simulink model "SPGF_FSK_0000_R2020b"  (R2020b)
settings: Solver=ode4  StartTime=0.0  StopTime=1.4  FixedStep=50e-6/50  RelTol=1e-3  EnableMultiTasking=on
undefined symbols (not defined in the file): D11, Delta
libraries: powerlib x2546, powerlib_meascontrol x183, simulink x24
(part 16 of 34)

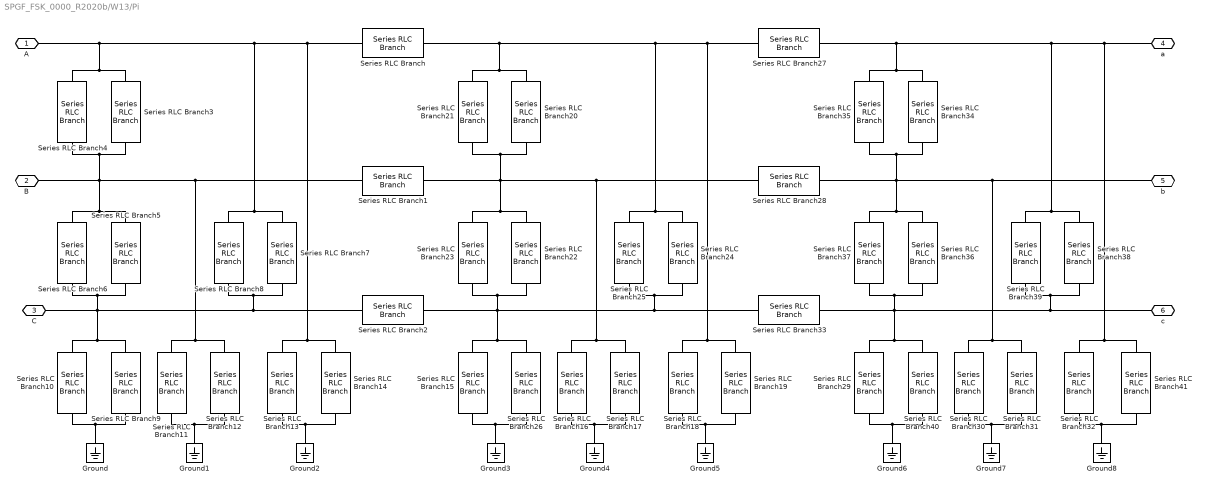
== system SPGF_FSK_0000_R2020b/W13/Pi ==
  Ground{,1..8} (9 alike) : powerlib/Elements/Ground  LConnTagsString=a
  Series RLC Branch{,1..2,27..28,33} (6 alike) : powerlib/Elements/Series RLC Branch  LConnTagsString=__new0  RConnTagsString=__new0  BranchType=RL  Resistance=R/2  Inductance=L/2  SetiL0=off  InitialCurrent=0  Capacitance=1e-6  Setx0=off  InitialVoltage=0  Measurements=None
  Series RLC Branch{10..11,13,29..30,32} (6 alike) : powerlib/Elements/Series RLC Branch  LConnTagsString=__new0  RConnTagsString=__new0  BranchType=R  Resistance=Rfg*4  Inductance=L/2  SetiL0=off  InitialCurrent=0  Capacitance=1e-6  Setx0=off  InitialVoltage=0  Measurements=None
  Series RLC Branch{9,12,14,31,40..41} (6 alike) : powerlib/Elements/Series RLC Branch  LConnTagsString=__new0  RConnTagsString=__new0  BranchType=C  Resistance=R/2  Inductance=L/2  SetiL0=off  InitialCurrent=0  Capacitance=Cfg*0.25  Setx0=off  InitialVoltage=0  Measurements=None
  Series RLC Branch15 : powerlib/Elements/Series RLC Branch  LConnTagsString=__new0  RConnTagsString=__new0  BranchType=R  Resistance=Rfg*2  Inductance=L/2  SetiL0=off  InitialCurrent=0  Capacitance=1e-6  Setx0=off  InitialVoltage=0  Measurements=None
  Series RLC Branch16 : powerlib/Elements/Series RLC Branch  LConnTagsString=__new0  RConnTagsString=__new0  BranchType=R  Resistance=Rfg*2  Inductance=L/2  SetiL0=off  InitialCurrent=0  Capacitance=1e-6  Setx0=off  InitialVoltage=0  Measurements=None
  Series RLC Branch17 : powerlib/Elements/Series RLC Branch  LConnTagsString=__new0  RConnTagsString=__new0  BranchType=C  Resistance=R/2  Inductance=L/2  SetiL0=off  InitialCurrent=0  Capacitance=Cfg*0.5  Setx0=off  InitialVoltage=0  Measurements=None
  Series RLC Branch18 : powerlib/Elements/Series RLC Branch  LConnTagsString=__new0  RConnTagsString=__new0  BranchType=R  Resistance=Rfg*2  Inductance=L/2  SetiL0=off  InitialCurrent=0  Capacitance=1e-6  Setx0=off  InitialVoltage=0  Measurements=None
  Series RLC Branch19 : powerlib/Elements/Series RLC Branch  LConnTagsString=__new0  RConnTagsString=__new0  BranchType=C  Resistance=R/2  Inductance=L/2  SetiL0=off  InitialCurrent=0  Capacitance=Cfg*0.5  Setx0=off  InitialVoltage=0  Measurements=None
  Series RLC Branch20 : powerlib/Elements/Series RLC Branch  LConnTagsString=__new0  RConnTagsString=__new0  BranchType=C  Resistance=R/2  Inductance=L/2  SetiL0=off  InitialCurrent=0  Capacitance=Cmf*0.5  Setx0=off  InitialVoltage=0  Measurements=None
  Series RLC Branch21 : powerlib/Elements/Series RLC Branch  LConnTagsString=__new0  RConnTagsString=__new0  BranchType=R  Resistance=Rmf*2  Inductance=L/2  SetiL0=off  InitialCurrent=0  Capacitance=1e-6  Setx0=off  InitialVoltage=0  Measurements=None
  Series RLC Branch22 : powerlib/Elements/Series RLC Branch  LConnTagsString=__new0  RConnTagsString=__new0  BranchType=C  Resistance=R/2  Inductance=L/2  SetiL0=off  InitialCurrent=0  Capacitance=Cmf*0.5  Setx0=off  InitialVoltage=0  Measurements=None
  Series RLC Branch23 : powerlib/Elements/Series RLC Branch  LConnTagsString=__new0  RConnTagsString=__new0  BranchType=R  Resistance=Rmf*2  Inductance=L/2  SetiL0=off  InitialCurrent=0  Capacitance=1e-6  Setx0=off  InitialVoltage=0  Measurements=None
  Series RLC Branch24 : powerlib/Elements/Series RLC Branch  LConnTagsString=__new0  RConnTagsString=__new0  BranchType=C  Resistance=R/2  Inductance=L/2  SetiL0=off  InitialCurrent=0  Capacitance=Cmf*0.5  Setx0=off  InitialVoltage=0  Measurements=None
  Series RLC Branch25 : powerlib/Elements/Series RLC Branch  LConnTagsString=__new0  RConnTagsString=__new0  BranchType=R  Resistance=Rmf*2  Inductance=L/2  SetiL0=off  InitialCurrent=0  Capacitance=1e-6  Setx0=off  InitialVoltage=0  Measurements=None
  Series RLC Branch26 : powerlib/Elements/Series RLC Branch  LConnTagsString=__new0  RConnTagsString=__new0  BranchType=C  Resistance=R/2  Inductance=L/2  SetiL0=off  InitialCurrent=0  Capacitance=Cfg*0.5  Setx0=off  InitialVoltage=0  Measurements=None
  Series RLC Branch{3,5,7,34,36,38} (6 alike) : powerlib/Elements/Series RLC Branch  LConnTagsString=__new0  RConnTagsString=__new0  BranchType=C  Resistance=R/2  Inductance=L/2  SetiL0=off  InitialCurrent=0  Capacitance=Cmf*0.25  Setx0=off  InitialVoltage=0  Measurements=None
  Series RLC Branch{4,6,8,35,37,39} (6 alike) : powerlib/Elements/Series RLC Branch  LConnTagsString=__new0  RConnTagsString=__new0  BranchType=R  Resistance=Rmf*4  Inductance=L/2  SetiL0=off  InitialCurrent=0  Capacitance=1e-6  Setx0=off  InitialVoltage=0  Measurements=None
  A : PMIOPort  Side=Left
  B : PMIOPort  Port=2  Side=Left
  C : PMIOPort  Port=3  Side=Left
  a : PMIOPort  Port=4  Side=Right
  b : PMIOPort  Port=5  Side=Right
  c : PMIOPort  Port=6  Side=Right
  connections:
  Ground8/LConn1 -- Series RLC Branch41/RConn1 -- Series RLC Branch32/RConn1
  Ground7/LConn1 -- Series RLC Branch30/RConn1 -- Series RLC Branch31/RConn1
  Ground6/LConn1 -- Series RLC Branch40/RConn1 -- Series RLC Branch29/RConn1
  Series RLC Branch40/LConn1 -- Series RLC Branch33/RConn1 -- Series RLC Branch38/RConn1 -- Series RLC Branch39/RConn1 -- c/RConn1 -- Series RLC Branch37/RConn1 -- Series RLC Branch36/RConn1 -- Series RLC Branch29/LConn1
  Series RLC Branch35/LConn1 -- Series RLC Branch27/RConn1 -- Series RLC Branch39/LConn1 -- Series RLC Branch38/LConn1 -- Series RLC Branch32/LConn1 -- Series RLC Branch41/LConn1 -- a/RConn1 -- Series RLC Branch34/LConn1
  Series RLC Branch30/LConn1 -- Series RLC Branch28/RConn1 -- Series RLC Branch37/LConn1 -- Series RLC Branch36/LConn1 -- Series RLC Branch34/RConn1 -- Series RLC Branch35/RConn1 -- b/RConn1 -- Series RLC Branch31/LConn1
  Series RLC Branch19/RConn1 -- Series RLC Branch18/RConn1 -- Ground5/LConn1
  Series RLC Branch16/RConn1 -- Series RLC Branch17/RConn1 -- Ground4/LConn1
  Ground3/LConn1 -- Series RLC Branch15/RConn1 -- Series RLC Branch26/RConn1
  Series RLC Branch23/RConn1 -- Series RLC Branch22/RConn1 -- Series RLC Branch24/RConn1 -- Series RLC Branch25/RConn1 -- Series RLC Branch33/LConn1 -- Series RLC Branch2/RConn1 -- Series RLC Branch15/LConn1 -- Series RLC Branch26/LConn1
  Series RLC Branch25/LConn1 -- Series RLC Branch24/LConn1 -- Series RLC Branch18/LConn1 -- Series RLC Branch19/LConn1 -- Series RLC Branch27/LConn1 -- Series RLC Branch/RConn1 -- Series RLC Branch20/LConn1 -- Series RLC Branch21/LConn1
  Series RLC Branch21/RConn1 -- Series RLC Branch20/RConn1 -- Series RLC Branch22/LConn1 -- Series RLC Branch23/LConn1 -- Series RLC Branch1/RConn1 -- Series RLC Branch28/LConn1 -- Series RLC Branch16/LConn1 -- Series RLC Branch17/LConn1
  Ground2/LConn1 -- Series RLC Branch14/RConn1 -- Series RLC Branch13/RConn1
  Ground1/LConn1 -- Series RLC Branch11/RConn1 -- Series RLC Branch12/RConn1
  Series RLC Branch10/RConn1 -- Ground/LConn1 -- Series RLC Branch9/RConn1
  Series RLC Branch10/LConn1 -- Series RLC Branch6/RConn1 -- Series RLC Branch5/RConn1 -- C/RConn1 -- Series RLC Branch7/RConn1 -- Series RLC Branch8/RConn1 -- Series RLC Branch2/LConn1 -- Series RLC Branch9/LConn1
  Series RLC Branch14/LConn1 -- Series RLC Branch/LConn1 -- Series RLC Branch8/LConn1 -- Series RLC Branch7/LConn1 -- Series RLC Branch3/LConn1 -- Series RLC Branch4/LConn1 -- A/RConn1 -- Series RLC Branch13/LConn1
  Series RLC Branch1/LConn1 -- Series RLC Branch3/RConn1 -- Series RLC Branch4/RConn1 -- B/RConn1 -- Series RLC Branch6/LConn1 -- Series RLC Branch5/LConn1 -- Series RLC Branch11/LConn1 -- Series RLC Branch12/LConn1

== system SPGF_FSK_0000_R2020b/W13/Q ==
  breaker : Subsystem  Commented=on  mask{SwitchA=off, SwitchB=off, SwitchC=off, InitialStatus=[1 1 1], BreakerResistance=0.0001, SnubberResistance=1e6, SnubberCapacitance=inf, TransitionTimes=[0.5 0.7], ShiftTimes=[0 0 0]}
      mask prompts: SwitchA "Switching of phase A"; SwitchB "Switching of phase B"; SwitchC "Switching of phase C"; InitialStatus "Initial status of phase breaker [A, B, C]"; BreakerResistance "Breaker resistance Ron (ohms) :"; SnubberResistance "Snubbers resistance Rp (ohms) :"; SnubberCapacitance "Snubbers capacitance Cp (F) :"; TransitionTimes "Transition times (s) :"; ShiftTimes "Time differences for switch [tA, tB, tC] (s) :"
      mask init: same as SPGF_FSK_0000_R2020b/Feed/Q/breaker
      mask Display:
      | % port_label('input',1,'Iabc');
      | 
      | port_label('lconn',1,'A');
      | port_label('lconn',2,'B');
      | port_label('lconn',3,'C');
      | 
      | port_label('rconn',1,'a');
      | port_label('rconn',2,'b');
      | port_label('rconn',3,'c');
      | 
      | disp('   Q    ');
  meas : Subsystem
  shunt : Subsystem
  A : PMIOPort  Side=Right
  B : PMIOPort  Port=2  Side=Right
  C : PMIOPort  Port=3  Side=Right
  a : PMIOPort  Port=4  Side=Left
  b : PMIOPort  Port=5  Side=Left
  c : PMIOPort  Port=6  Side=Left
  connections:
  shunt/LConn3 -- C/RConn1 -- breaker/LConn3
  shunt/LConn2 -- B/RConn1 -- breaker/LConn2
  A/RConn1 -- shunt/LConn1 -- breaker/LConn1
  meas/RConn1 -- a/RConn1
  meas/RConn2 -- b/RConn1
  meas/RConn3 -- c/RConn1
  meas/LConn3 -- breaker/RConn3 -- shunt/RConn3
  meas/LConn2 -- breaker/RConn2 -- shunt/RConn2
  meas/LConn1 -- breaker/RConn1 -- shunt/RConn1

== system SPGF_FSK_0000_R2020b/W13/concentrated ==
  Ccs/1 : powerlib/Elements/Series RLC Branch  LConnTagsString=__new0  RConnTagsString=__new0  BranchType=C  Resistance=190  Inductance=1e-3  SetiL0=off  InitialCurrent=0  Capacitance=-C_matrix(1,2)/2  Setx0=off  InitialVoltage=0  Measurements=None
  Ccs/2 : powerlib/Elements/Series RLC Branch  LConnTagsString=__new0  RConnTagsString=__new0  BranchType=C  Resistance=190  Inductance=1e-3  SetiL0=off  InitialCurrent=0  Capacitance=-C_matrix(1,2)/2  Setx0=off  InitialVoltage=0  Measurements=None
  Ccs2/1 : powerlib/Elements/Series RLC Branch  LConnTagsString=__new0  RConnTagsString=__new0  BranchType=C  Resistance=190  Inductance=1e-3  SetiL0=off  InitialCurrent=0  Capacitance=-C_matrix(3,4)/2  Setx0=off  InitialVoltage=0  Measurements=None
  Ccs2/2 : powerlib/Elements/Series RLC Branch  LConnTagsString=__new0  RConnTagsString=__new0  BranchType=C  Resistance=190  Inductance=1e-3  SetiL0=off  InitialCurrent=0  Capacitance=-C_matrix(3,4)/2  Setx0=off  InitialVoltage=0  Measurements=None
  Ccs2/3 : powerlib/Elements/Series RLC Branch  LConnTagsString=__new0  RConnTagsString=__new0  BranchType=R  Resistance=-Rg_matrix(3,4)*2  Inductance=1e-3  SetiL0=off  InitialCurrent=0  Capacitance=Rg_matrix(3,4)*2  Setx0=off  InitialVoltage=0  Measurements=None
  Ccs2/4 : powerlib/Elements/Series RLC Branch  LConnTagsString=__new0  RConnTagsString=__new0  BranchType=R  Resistance=-Rg_matrix(3,4)*2  Inductance=1e-3  SetiL0=off  InitialCurrent=0  Capacitance=Rg_matrix(3,4)*2  Setx0=off  InitialVoltage=0  Measurements=None
  Ccs3/1 : powerlib/Elements/Series RLC Branch  LConnTagsString=__new0  RConnTagsString=__new0  BranchType=C  Resistance=190  Inductance=1e-3  SetiL0=off  InitialCurrent=0  Capacitance=-C_matrix(5,6)/2  Setx0=off  InitialVoltage=0  Measurements=None
  Ccs3/2 : powerlib/Elements/Series RLC Branch  LConnTagsString=__new0  RConnTagsString=__new0  BranchType=C  Resistance=190  Inductance=1e-3  SetiL0=off  InitialCurrent=0  Capacitance=-C_matrix(5,6)/2  Setx0=off  InitialVoltage=0  Measurements=None
  Ccs3/3 : powerlib/Elements/Series RLC Branch  LConnTagsString=__new0  RConnTagsString=__new0  BranchType=R  Resistance=-Rg_matrix(5,6)*2  Inductance=1e-3  SetiL0=off  InitialCurrent=0  Capacitance=-C_matrix(5,6)/2  Setx0=off  InitialVoltage=0  Measurements=None
  Ccs3/4 : powerlib/Elements/Series RLC Branch  LConnTagsString=__new0  RConnTagsString=__new0  BranchType=R  Resistance=-Rg_matrix(5,6)*2  Inductance=1e-3  SetiL0=off  InitialCurrent=0  Capacitance=-C_matrix(5,6)/2  Setx0=off  InitialVoltage=0  Measurements=None
  Csg/2 : powerlib/Elements/Series RLC Branch  LConnTagsString=__new0  RConnTagsString=__new0  BranchType=C  Resistance=190  Inductance=1e-3  SetiL0=off  InitialCurrent=0  Capacitance=( C_matrix(1,2) + C_matrix(2,2) )/2  Setx0=off  InitialVoltage=0  Measurements=None
  Csg1/1 : powerlib/Elements/Series RLC Branch  LConnTagsString=__new0  RConnTagsString=__new0  BranchType=C  Resistance=190  Inductance=1e-3  SetiL0=off  InitialCurrent=0  Capacitance=( C_matrix(1,2) + C_matrix(2,2) )/2  Setx0=off  InitialVoltage=0  Measurements=None
  Csg2/1 : powerlib/Elements/Series RLC Branch  LConnTagsString=__new0  RConnTagsString=__new0  BranchType=C  Resistance=190  Inductance=1e-3  SetiL0=off  InitialCurrent=0  Capacitance=( C_matrix(3,4) + C_matrix(4,4) )/2  Setx0=off  InitialVoltage=0  Measurements=None
  Csg2/2 : powerlib/Elements/Series RLC Branch  LConnTagsString=__new0  RConnTagsString=__new0  BranchType=C  Resistance=190  Inductance=1e-3  SetiL0=off  InitialCurrent=0  Capacitance=( C_matrix(3,4) + C_matrix(4,4) )/2  Setx0=off  InitialVoltage=0  Measurements=None
  Csg3/1 : powerlib/Elements/Series RLC Branch  LConnTagsString=__new0  RConnTagsString=__new0  BranchType=C  Resistance=190  Inductance=1e-3  SetiL0=off  InitialCurrent=0  Capacitance=( C_matrix(5,6) + C_matrix(6,6) ) /2  Setx0=off  InitialVoltage=0  Measurements=None
  Csg3/2 : powerlib/Elements/Series RLC Branch  LConnTagsString=__new0  RConnTagsString=__new0  BranchType=C  Resistance=190  Inductance=1e-3  SetiL0=off  InitialCurrent=0  Capacitance=( C_matrix(5,6) + C_matrix(6,6) ) /2  Setx0=off  InitialVoltage=0  Measurements=None
  Ground{1..4} (4 alike) : powerlib/Elements/Ground  LConnTagsString=a
  RL : powerlib/Elements/Mutual Inductance  LConnTagsString=a|b|c|L4|L5|L6  RConnTagsString=A|B|C|R4|R5|R6  TypeOfMutual=Generalized mutual inductance  NumberOfWindings=6  SelfImpedance1=[1.1 1.1e-03]  SelfImpedance2=[ 1.1 1.1e-03]  ThreeWindings=on  SelfImpedance3=[ 1.1 1.1e-03]  MutualImpedance=[1.0 1.0e-03]  InductanceMatrix=L_matrix  ResistanceMatrix=R_matrix  Measurements=None
      settings: AttributesFormatString=\n
  Rcs*2 : powerlib/Elements/Series RLC Branch  LConnTagsString=__new0  RConnTagsString=__new0  BranchType=R  Resistance=-Rg_matrix(1,2)*2  Inductance=1e-3  SetiL0=off  InitialCurrent=0  Capacitance=Rg_matrix(1,2)*2  Setx0=off  InitialVoltage=0  Measurements=None
  Rgcs1/1 : powerlib/Elements/Series RLC Branch  LConnTagsString=__new0  RConnTagsString=__new0  BranchType=R  Resistance=-Rg_matrix(1,2)*2  Inductance=1e-3  SetiL0=off  InitialCurrent=0  Capacitance=Rg_matrix(1,2)*2  Setx0=off  InitialVoltage=0  Measurements=None
  Rgsg1/1 : powerlib/Elements/Series RLC Branch  LConnTagsString=__new0  RConnTagsString=__new0  BranchType=R  Resistance=(Rg_matrix(4,4)+Rg_matrix(3,4))*2  Inductance=1e-3  SetiL0=off  InitialCurrent=0  Capacitance=Rg_matrix(1,2)*2  Setx0=off  InitialVoltage=0  Measurements=None
  Rgsg1/2 : powerlib/Elements/Series RLC Branch  LConnTagsString=__new0  RConnTagsString=__new0  BranchType=R  Resistance=(Rg_matrix(2,2)+Rg_matrix(1,2))*2  Inductance=1e-3  SetiL0=off  InitialCurrent=0  Capacitance=Rg_matrix(1,2)*2  Setx0=off  InitialVoltage=0  Measurements=None
  Rgsg1/3 : powerlib/Elements/Series RLC Branch  LConnTagsString=__new0  RConnTagsString=__new0  BranchType=R  Resistance=(Rg_matrix(4,4)+Rg_matrix(3,4))*2  Inductance=1e-3  SetiL0=off  InitialCurrent=0  Capacitance=Rg_matrix(1,2)*2  Setx0=off  InitialVoltage=0  Measurements=None
  Rgsg1/4 : powerlib/Elements/Series RLC Branch  LConnTagsString=__new0  RConnTagsString=__new0  BranchType=R  Resistance=(Rg_matrix(2,2)+Rg_matrix(1,2))*2  Inductance=1e-3  SetiL0=off  InitialCurrent=0  Capacitance=Rg_matrix(1,2)*2  Setx0=off  InitialVoltage=0  Measurements=None
  Rsg*2 : powerlib/Elements/Series RLC Branch  LConnTagsString=__new0  RConnTagsString=__new0  BranchType=R  Resistance=(Rg_matrix(6,6)+Rg_matrix(5,6))*2  Inductance=1e-3  SetiL0=off  InitialCurrent=0  Capacitance=Rg_matrix(1,2)*2  Setx0=off  InitialVoltage=0  Measurements=None
  Rsg1/1 : powerlib/Elements/Series RLC Branch  LConnTagsString=__new0  RConnTagsString=__new0  BranchType=R  Resistance=(Rg_matrix(6,6)+Rg_matrix(5,6))*2  Inductance=1e-3  SetiL0=off  InitialCurrent=0  Capacitance=Rg_matrix(1,2)*2  Setx0=off  InitialVoltage=0  Measurements=None
  A : PMIOPort  Side=Left
  B : PMIOPort  Port=2  Side=Left
  C : PMIOPort  Port=3  Side=Left
  a : PMIOPort  Port=4  Side=Right
  b : PMIOPort  Port=5  Side=Right
  c : PMIOPort  Port=6  Side=Right
  connections:
  Ccs3/3/RConn1 -- RL/LConn5 -- C/RConn1 -- Ccs3/2/RConn1
  Ccs2/2/RConn1 -- Ccs2/3/RConn1 -- B/RConn1 -- RL/LConn3
  Ccs/2/RConn1 -- Rcs*2/RConn1 -- A/RConn1 -- RL/LConn1
  Ccs3/4/RConn1 -- RL/RConn5 -- c/RConn1 -- Ccs3/1/RConn1
  Ccs2/1/RConn1 -- Ccs2/4/RConn1 -- RL/RConn3 -- b/RConn1
  Ccs/1/RConn1 -- Rgcs1/1/RConn1 -- RL/RConn1 -- a/RConn1
  Csg/2/RConn1 -- Ground1/LConn1 -- Csg2/2/RConn1 -- Csg3/2/RConn1 -- Rgsg1/2/RConn1 -- Rgsg1/1/RConn1 -- Rsg*2/RConn1
  Csg3/1/LConn1 -- Ccs3/4/LConn1 -- Rsg1/1/LConn1 -- Ccs3/1/LConn1 -- RL/RConn6 -- Ground4/LConn1 -- RL/RConn2 -- Ccs/1/LConn1 -- Csg1/1/LConn1 -- Rgcs1/1/LConn1 -- Rgsg1/4/LConn1 -- RL/RConn4 -- Ccs2/1/LConn1 -- Csg2/1/LConn1 -- Ccs2/4/LConn1 -- Rgsg1/3/LConn1
  Csg1/1/RConn1 -- Ground2/LConn1 -- Csg2/1/RConn1 -- Csg3/1/RConn1 -- Rgsg1/4/RConn1 -- Rgsg1/3/RConn1 -- Rsg1/1/RConn1
  Ccs3/2/LConn1 -- Ccs3/3/LConn1 -- Csg3/2/LConn1 -- Rsg*2/LConn1 -- Ccs2/2/LConn1 -- Ccs2/3/LConn1 -- Csg2/2/LConn1 -- Rgsg1/1/LConn1 -- RL/LConn4 -- RL/LConn2 -- Ccs/2/LConn1 -- Rcs*2/LConn1 -- Csg/2/LConn1 -- Rgsg1/2/LConn1 -- Ground3/LConn1 -- RL/LConn6

== system SPGF_FSK_0000_R2020b/W14/DPL ==
  Ccs2/1 : powerlib/Elements/Series RLC Branch  LConnTagsString=__new0  RConnTagsString=__new0  BranchType=R  Resistance=-Rg_matrix(3,4)*2  Inductance=1e-3  SetiL0=off  InitialCurrent=0  Capacitance=Rg_matrix(3,4)*2  Setx0=off  InitialVoltage=0  Measurements=None
  Ccs2/3 : powerlib/Elements/Series RLC Branch  LConnTagsString=__new0  RConnTagsString=__new0  BranchType=R  Resistance=-Rg_matrix(3,4)*2  Inductance=1e-3  SetiL0=off  InitialCurrent=0  Capacitance=Rg_matrix(3,4)*2  Setx0=off  InitialVoltage=0  Measurements=None
  Ccs3/1 : powerlib/Elements/Series RLC Branch  LConnTagsString=__new0  RConnTagsString=__new0  BranchType=R  Resistance=-Rg_matrix(5,6)*2  Inductance=1e-3  SetiL0=off  InitialCurrent=0  Capacitance=-C_matrix(5,6)/2  Setx0=off  InitialVoltage=0  Measurements=None
  Ccs3/3 : powerlib/Elements/Series RLC Branch  LConnTagsString=__new0  RConnTagsString=__new0  BranchType=R  Resistance=-Rg_matrix(5,6)*2  Inductance=1e-3  SetiL0=off  InitialCurrent=0  Capacitance=-C_matrix(5,6)/2  Setx0=off  InitialVoltage=0  Measurements=None
  DPL : powerlib/Elements/Distributed Parameters Line  Phases=6  Length=LineLength  Frequency=Frequency  Resistance=R_matrix  Inductance=L_matrix  Capacitance=C_matrix  x1=[-2.8e-05 -0.96563974701064 4525.01977205028 -12.1288151005584 -2553.87771291034 0 0;-2.75e-05 -0.965894057806881 4526.29000191823 -12.1318920997408 -2554.59461845184 0 0;-2.7e-05 -0.966148344770642 4527.56012010445 -12.1349687995808 -2555.31146096124 0 0;-2.65e-05 -0.966402607895648 4528.83012657761 -12.1380452000024 -2556.02824042086 0 0;-2.6e-05 -0.966656847175625 4530.10002130636 -12.1411213009297 -2556.74495681301 0 0;-2.55e-05 -0.9669110626043 4531.36980425937 -12.1441971022869 -2557.46161012001 0 0;-2.5e-05 -0.967165254175402 4532.63947540531 -12.1472726039981 -2558.17820032417 0 0;-2.45e-05 -0.967419421882657 4533.90903471286 -12.1503478059873 -2558.89472740782 0 0;-2.4e-05 -0.967673565719795 4535.17848215069 -12.1534227081787 -2559.61119135326 0 0;-2.35e-05 -0.967927685680545 4536.44781768747 -12.1564973104964 -2560.32759214284 0 0;-2.3e-05 -0.968181781758636 4537.71704129189 -12.1595716128645 -2561.04392975886 0 0;-2.25e-05 -0.9684358539478 4538.98615293264 -12.1626456152073 -2561.76020418365 0 0;-2.2e-05 -0.968689902241767 4540.25515257838 -12.1657193174488 -2562.47641539955 0 0;-2.15e-05 -0.968943926634268 4541.52404019782 -12.1687927195132 -2563.19256338888 0 0;-2.1e-05 -0.969197927119037 4542.79281575965 -12.1718658213247 -2563.90864813396 0 0;-2.05e-05 -0.969451903689805 4544.06147923256 -12.1749386228074 -2564.62466961714 0 0;-2e-05 -0.969705856340306 4545.33003058525 -12.1780111238856 -2565.34062782073 0 0;-1.95e-05 -0.969959785064274 4546.59846978641 -12.1810833244834 -2566.05652272709 0 0;-1.9e-05 -0.970213689855444 4547.86679680475 -12.184155224525 -2566.77235431853 0 0;-1.85e-05 -0.970467570707551 4549.13501160898 -12.1872268239346 -2567.48812257741 0 0;-1.8e-05 -0.97072142761433 4550.4031141678 -12.1902981226365 -2568.20382748606 0 0;-1.75e-05 -0.970975260569519 4551.67110444992 -12.1933691205548 -2568.91946902682 0 0;-1.7e-05 -0.971229069566853 4552.93898242406 -12.1964398176138 -2569.63504718203 0 0;-1.65e-05 -0.97148285460007 4554.20674805893 -12.1995102137377 -2570.35056193404 0 0;-1.6e-05 -0.971736615662908 4555.47440132326 -12.2025803088507 -2571.06601326519 0 0;-1.55e-05 -0.971990352749107 4556.74194218576 -12.2056501028772 -2571.78140115783 0 0;-1.5e-05 -0.972244065852405 4558.00937061516 -12.2087195957413 -2572.49672559431 0 0;-1.45e-05 -0.972497754966543 4559.27668658019 -12.2117887873673 -2573.21198655697 0 0;-1.4e-05 -0.97275142008526 4560.54389004958 -12.2148576776795 -2573.92718402818 0 0;-1.35e-05 -0.973005061202298 4561.81098099205 -12.2179262666022 -2574.64231799027 0 0;-1.3e-05 -0.973258678311398 4563.07795937635 -12.2209945540596 -2575.35738842562 0 0;-1.25e-05 -0.973512271406303 4564.34482517122 -12.2240625399761 -2576.07239531657 0 0;-1.2e-05 -0.973765840480756 4565.61157834539 -12.2271302242759 -2576.78733864547 0 0;-1.15e-05 -0.9740193855285 4566.87821886761 -12.2301976068834 -2577.5022183947 0 0;-1.1e-05 -0.974272906543279 4568.14474670663 -12.2332646877229 -2578.21703454662 0 0;-1.05e-05 -0.974526403518837 4569.41116183119 -12.2363314667186 -2578.93178708357 0 0;-1e-05 -0.97477987644892 4570.67746421006 -12.239397943795 -2579.64647598794 0 0;-9.5e-06 -0.975033325327274 4571.94365381198 -12.2424641188763 -2580.36110124208 0 0;-9e-06 -0.975286750147645 4573.20973060571 -12.2455299918869 -2581.07566282836 0 0;-8.5e-06 -0.97554015090378 4574.47569456001 -12.2485955627512 -2581.79016072915 0 0;-8e-06 -0.975793527589426 4575.74154564365 -12.2516608313935 -2582.50459492683 0 0;-7.5e-06 -0.976046880198333 4577.00728382539 -12.2547257977382 -2583.21896540376 0 0;-7e-06 -0.976300208724248 4578.27290907401 -12.2577904617097 -2583.93327214231 0 0;-6.5e-06 -0.976553513160921 4579.53842135826 -12.2608548232323 -2584.64751512487 0 0;-6e-06 -0.976806793502102 4580.80382064694 -12.2639188822304 -2585.3616943338 0 0;-5.5e-06 -0.977060049741541 4582.06910690882 -12.2669826386285 -2586.07580975149 0 0;-5e-06 -0.97731328187299 4583.33428011267 -12.2700460923509 -2586.78986136032 0 0;-4.5e-06 ...(+1014 chars)]  x2=[-2.8e-05 -0.965202073515616 4526.4078296794 -12.1181827595672 -2554.66111930831 0 0;-2.75e-05 -0.965457756270191 4527.68150549754 -12.1212814453172 -2555.37996971101 0 0;-2.7e-05 -0.965713415203051 4528.95506959962 -12.1243798319867 -2556.09875706224 0 0;-2.65e-05 -0.965969050307887 4530.22852195421 -12.127477919499 -2556.81748134425 0 0;-2.6e-05 -0.966224661578392 4531.5018625299 -12.1305757077778 -2557.53614253933 0 0;-2.55e-05 -0.96648024900826 4532.77509129525 -12.1336731967467 -2558.25474062973 0 0;-2.5e-05 -0.966735812591183 4534.04820821886 -12.1367703863292 -2558.97327559772 0 0;-2.45e-05 -0.966991352320856 4535.32121326932 -12.1398672764489 -2559.69174742558 0 0;-2.4e-05 -0.967246868190974 4536.59410641522 -12.1429638670294 -2560.41015609558 0 0;-2.35e-05 -0.967502360195232 4537.86688762514 -12.1460601579942 -2561.12850158999 0 0;-2.3e-05 -0.967757828327326 4539.13955686768 -12.149156149267 -2561.84678389108 0 0;-2.25e-05 -0.968013272580953 4540.41211411145 -12.1522518407714 -2562.56500298114 0 0;-2.2e-05 -0.96826869294981 4541.68455932503 -12.155347232431 -2563.28315884245 0 0;-2.15e-05 -0.968524089427594 4542.95689247704 -12.1584423241695 -2564.00125145727 0 0;-2.1e-05 -0.968779462008005 4544.22911353609 -12.1615371159104 -2564.71928080791 0 0;-2.05e-05 -0.96903481068474 4545.50122247077 -12.1646316075774 -2565.43724687663 0 0;-2e-05 -0.9692901354515 4546.77321924971 -12.1677257990941 -2566.15514964572 0 0;-1.95e-05 -0.969545436301985 4548.04510384152 -12.1708196903843 -2566.87298909747 0 0;-1.9e-05 -0.969800713229895 4549.31687621481 -12.1739132813715 -2567.59076521417 0 0;-1.85e-05 -0.970055966228931 4550.5885363382 -12.1770065719794 -2568.30847797811 0 0;-1.8e-05 -0.970311195292796 4551.86008418033 -12.1800995621318 -2569.02612737158 0 0;-1.75e-05 -0.970566400415192 4553.13151970981 -12.1831922517522 -2569.74371337687 0 0;-1.7e-05 -0.970821581589822 4554.40284289527 -12.1862846407644 -2570.46123597627 0 0;-1.65e-05 -0.971076738810389 4555.67405370535 -12.1893767290921 -2571.17869515209 0 0;-1.6e-05 -0.971331872070598 4556.94515210867 -12.192468516659 -2571.89609088661 0 0;-1.55e-05 -0.971586981364155 4558.21613807388 -12.1955600033888 -2572.61342316214 0 0;-1.5e-05 -0.971842066684763 4559.48701156962 -12.1986511892052 -2573.33069196098 0 0;-1.45e-05 -0.972097128026129 4560.75777256452 -12.2017420740319 -2574.04789726543 0 0;-1.4e-05 -0.972352165381961 4562.02842102724 -12.2048326577928 -2574.7650390578 0 0;-1.35e-05 -0.972607178745964 4563.29895692641 -12.2079229404114 -2575.48211732038 0 0;-1.3e-05 -0.972862168111847 4564.5693802307 -12.2110129218116 -2576.19913203549 0 0;-1.25e-05 -0.973117133473319 4565.83969090876 -12.2141026019172 -2576.91608318543 0 0;-1.2e-05 -0.973372074824087 4567.10988892923 -12.2171919806519 -2577.63297075252 0 0;-1.15e-05 -0.973626992157863 4568.37997426079 -12.2202810579394 -2578.34979471906 0 0;-1.1e-05 -0.973881885468355 4569.64994687208 -12.2233698337036 -2579.06655506738 0 0;-1.05e-05 -0.974136754749275 4570.91980673179 -12.2264583078682 -2579.78325177977 0 0;-1e-05 -0.974391599994334 4572.18955380857 -12.2295464803571 -2580.49988483857 0 0;-9.5e-06 -0.974646421197244 4573.45918807109 -12.232634351094 -2581.21645422608 0 0;-9e-06 -0.974901218351717 4574.72870948804 -12.2357219200027 -2581.93295992463 0 0;-8.5e-06 -0.975155991451468 4575.99811802807 -12.2388091870071 -2582.64940191654 0 0;-8e-06 -0.975410740490208 4577.26741365988 -12.241896152031 -2583.36578018413 0 0;-7.5e-06 -0.975665465461653 4578.53659635214 -12.2449828149982 -2584.08209470972 0 0;-7e-06 -0.975920166359518 4579.80566607354 -12.2480691758326 -2584.79834547565 0 0;-6.5e-06 -0.976174843177518 4581.07462279277 -12.2511552344579 -2585.51453246423 0 0;-6e-06 -0.97642949590937 4582.34346647851 -12.2542409907982 -2586.2306556578 0 0;-5.5e-06 -0.976684124548789 4583.61219709945 -12.2573264447771 -2586.94671503868 0 0;-5e-06 -0.976938729089493 4584.8808146243 -12.2604115963187 -2587.66271058921 0 0;-4.5e-06 ...(+1007 chars)]  x3=[-2.8e-05 -0.000381042548598165 39.2393208593552 -0.539758671733172 -178.575955753185 0 0;-2.75e-05 -0.000382787670081508 39.2600914589651 -0.539953528025206 -178.629936562073 0 0;-2.7e-05 -0.000384532782119944 39.280861089871 -0.54014837099442 -178.683912963444 0 0;-2.65e-05 -0.000386277884670414 39.3016297515605 -0.540343200636007 -178.737884955967 0 0;-2.6e-05 -0.000388022977689859 39.3223974435212 -0.540538016945161 -178.791852538309 0 0;-2.55e-05 -0.000389768061135221 39.3431641652407 -0.540732819917073 -178.845815709139 0 0;-2.5e-05 -0.000391513134963442 39.3639299162064 -0.540927609546938 -178.899774467125 0 0;-2.45e-05 -0.000393258199131463 39.3846946959061 -0.541122385829949 -178.953728810936 0 0;-2.4e-05 -0.000395003253596227 39.4054585038275 -0.5413171487613 -179.007678739241 0 0;-2.35e-05 -0.000396748298314677 39.4262213394581 -0.541511898336187 -179.061624250709 0 0;-2.3e-05 -0.000398493333243755 39.4469832022857 -0.541706634549802 -179.115565344008 0 0;-2.25e-05 -0.000400238358340403 39.467744091798 -0.541901357397342 -179.169502017808 0 0;-2.2e-05 -0.000401983373561567 39.4885040074828 -0.542096066874003 -179.223434270777 0 0;-2.15e-05 -0.000403728378864187 39.5092629488277 -0.542290762974978 -179.277362101586 0 0;-2.1e-05 -0.00040547337420521 39.5300209153207 -0.542485445695466 -179.331285508903 0 0;-2.05e-05 -0.000407218359541578 39.5507779064496 -0.542680115030662 -179.385204491397 0 0;-2e-05 -0.000408963334830236 39.571533921702 -0.542874770975763 -179.43911904774 0 0;-1.95e-05 -0.000410708300028128 39.5922889605661 -0.543069413525965 -179.493029176599 0 0;-1.9e-05 -0.000412453255092199 39.6130430225295 -0.543264042676467 -179.546934876646 0 0;-1.85e-05 -0.000414198199979394 39.6337961070803 -0.543458658422466 -179.600836146549 0 0;-1.8e-05 -0.000415943134646658 39.6545482137064 -0.543653260759161 -179.65473298498 0 0;-1.75e-05 -0.000417688059050936 39.6752993418958 -0.543847849681748 -179.708625390607 0 0;-1.7e-05 -0.000419432973149175 39.6960494911363 -0.544042425185428 -179.762513362102 0 0;-1.65e-05 -0.000421177876898319 39.7167986609161 -0.544236987265399 -179.816396898135 0 0;-1.6e-05 -0.000422922770255317 39.7375468507232 -0.544431535916861 -179.870275997376 0 0;-1.55e-05 -0.000424667653177113 39.7582940600456 -0.544626071135013 -179.924150658496 0 0;-1.5e-05 -0.000426412525620655 39.7790402883714 -0.544820592915056 -179.978020880165 0 0;-1.45e-05 -0.00042815738754289 39.7997855351887 -0.545015101252189 -180.031886661055 0 0;-1.4e-05 -0.000429902238900764 39.8205297999858 -0.545209596141613 -180.085747999836 0 0;-1.35e-05 -0.000431647079651226 39.8412730822506 -0.54540407757853 -180.13960489518 0 0;-1.3e-05 -0.000433391909751224 39.8620153814714 -0.545598545558141 -180.193457345756 0 0;-1.25e-05 -0.000435136729157704 39.8827566971364 -0.545793000075648 -180.247305350238 0 0;-1.2e-05 -0.000436881537827616 39.9034970287338 -0.545987441126252 -180.301148907295 0 0;-1.15e-05 -0.000438626335717908 39.9242363757519 -0.546181868705155 -180.3549880156 0 0;-1.1e-05 -0.00044037112278553 39.944974737679 -0.546376282807562 -180.408822673824 0 0;-1.05e-05 -0.000442115898987429 39.9657121140033 -0.546570683428674 -180.462652880639 0 0;-1e-05 -0.000443860664280556 39.9864485042132 -0.546765070563695 -180.516478634716 0 0;-9.5e-06 -0.00044560541862186 40.007183907797 -0.546959444207828 -180.570299934727 0 0;-9e-06 -0.000447350161968291 40.0279183242431 -0.547153804356279 -180.624116779345 0 0;-8.5e-06 -0.000449094894276799 40.04865175304 -0.54734815100425 -180.677929167242 0 0;-8e-06 -0.000450839615504334 40.0693841936759 -0.547542484146947 -180.73173709709 0 0;-7.5e-06 -0.000452584325607849 40.0901156456395 -0.547736803779575 -180.78554056756 0 0;-7e-06 -0.000454329024544292 40.1108461084191 -0.547931109897339 -180.839339577326 0 0;-6.5e-06 -0.000456073712270616 40.1315755815032 -0.548125402495445 -180.893134125061 0 0;-6e-06 -0.000457818388743773 40.1523040643804 -0.548319681569098 -180.946924209436 0 0;-5.5e-06 ...(+1222 chars)]  x4=[-2.8e-05 -0.0107699366000144 58.8450264477869 -0.632850505385285 -177.531959493093 0 0;-2.75e-05 -0.0107711663063993 58.8518695391916 -0.632954946327498 -177.578233875616 0 0;-2.7e-05 -0.0107723957470163 58.8587111784847 -0.633059371652174 -177.624503876573 0 0;-2.65e-05 -0.010773624921835 58.8655513654973 -0.633163781356736 -177.67076949482 0 0;-2.6e-05 -0.0107748538308253 58.8723901000607 -0.633268175438607 -177.717030729217 0 0;-2.55e-05 -0.0107760824739566 58.8792273820061 -0.633372553895213 -177.763287578622 0 0;-2.5e-05 -0.0107773108511988 58.8860632111647 -0.633476916723977 -177.809540041894 0 0;-2.45e-05 -0.0107785389625215 58.892897587368 -0.633581263922326 -177.855788117891 0 0;-2.4e-05 -0.0107797668078944 58.8997305104473 -0.633685595487682 -177.902031805473 0 0;-2.35e-05 -0.0107809943872873 58.906561980234 -0.633789911417474 -177.948271103498 0 0;-2.3e-05 -0.0107822217006697 58.9133919965595 -0.633894211709127 -177.994506010825 0 0;-2.25e-05 -0.0107834487480115 58.9202205592553 -0.633998496360066 -178.040736526314 0 0;-2.2e-05 -0.0107846755292824 58.927047668153 -0.63410276536772 -178.086962648824 0 0;-2.15e-05 -0.0107859020444521 58.9338733230841 -0.634207018729516 -178.133184377214 0 0;-2.1e-05 -0.0107871282934903 58.9406975238801 -0.63431125644288 -178.179401710344 0 0;-2.05e-05 -0.0107883542763667 58.9475202703727 -0.634415478505241 -178.225614647073 0 0;-2e-05 -0.0107895799930513 58.9543415623936 -0.634519684914028 -178.271823186262 0 0;-1.95e-05 -0.0107908054435135 58.9611613997744 -0.63462387566667 -178.31802732677 0 0;-1.9e-05 -0.0107920306277234 58.9679797823468 -0.634728050760595 -178.364227067457 0 0;-1.85e-05 -0.0107932555456505 58.9747967099427 -0.634832210193233 -178.410422407182 0 0;-1.8e-05 -0.0107944801972648 58.9816121823938 -0.634936353962014 -178.456613344808 0 0;-1.75e-05 -0.0107957045825359 58.9884261995319 -0.635040482064369 -178.502799879193 0 0;-1.7e-05 -0.0107969287014337 58.995238761189 -0.635144594497727 -178.548982009197 0 0;-1.65e-05 -0.010798152553928 59.0020498671969 -0.635248691259521 -178.595159733682 0 0;-1.6e-05 -0.0107993761399885 59.0088595173875 -0.635352772347182 -178.641333051509 0 0;-1.55e-05 -0.0108005994595851 59.015667711593 -0.635456837758142 -178.687501961537 0 0;-1.5e-05 -0.0108018225126876 59.0224744496452 -0.635560887489833 -178.733666462628 0 0;-1.45e-05 -0.0108030452992658 59.0292797313762 -0.635664921539687 -178.779826553642 0 0;-1.4e-05 -0.0108042678192896 59.0360835566181 -0.635768939905138 -178.825982233441 0 0;-1.35e-05 -0.0108054900727287 59.0428859252031 -0.63587294258362 -178.872133500885 0 0;-1.3e-05 -0.010806712059553 59.0496868369632 -0.635976929572565 -178.918280354837 0 0;-1.25e-05 -0.0108079337797325 59.0564862917307 -0.636080900869409 -178.964422794157 0 0;-1.2e-05 -0.0108091552332368 59.0632842893378 -0.636184856471585 -179.010560817707 0 0;-1.15e-05 -0.0108103764200359 59.0700808296168 -0.63628879637653 -179.056694424348 0 0;-1.1e-05 -0.0108115973400997 59.0768759124 -0.636392720581678 -179.102823612943 0 0;-1.05e-05 -0.010812817993398 59.0836695375197 -0.636496629084464 -179.148948382352 0 0;-1e-05 -0.0108140383799007 59.0904617048083 -0.636600521882326 -179.195068731439 0 0;-9.5e-06 -0.0108152584995777 59.0972524140982 -0.6367043989727 -179.241184659064 0 0;-9e-06 -0.0108164783523989 59.1040416652218 -0.636808260353023 -179.28729616409 0 0;-8.5e-06 -0.0108176979383342 59.1108294580117 -0.636912106020731 -179.33340324538 0 0;-8e-06 -0.0108189172573535 59.1176157923003 -0.637015935973263 -179.379505901795 0 0;-7.5e-06 -0.0108201363094268 59.1244006679202 -0.637119750208057 -179.425604132198 0 0;-7e-06 -0.0108213550945238 59.131184084704 -0.637223548722551 -179.471697935452 0 0;-6.5e-06 -0.0108225736126146 59.1379660424843 -0.637327331514185 -179.51778731042 0 0;-6e-06 -0.0108237918636692 59.1447465410938 -0.637431098580397 -179.563872255963 0 0;-5.5e-06 -0.0108250098476573 59.1515255803652 -0.637534849918627 -179.609952770946 0 0;-5e-06 ...(+1122 chars)]  x5=2.77990901432774e-05  V1=ones(3,3)  V2=ones(3,3)  I1=ones(3,3)  I2=ones(3,3)  nHarmo=1  Measurements=None  Decoupling=off  VsMag0=0  VrMag0=0  VsAngle0=0  VrAngle0=0  IsMag0=0  IrMag0=0  IsAngle0=0  IrAngle0=0
  Ground{1..4} (4 alike) : powerlib/Elements/Ground  LConnTagsString=a
  Rcs*1 : powerlib/Elements/Series RLC Branch  LConnTagsString=__new0  RConnTagsString=__new0  BranchType=R  Resistance=-Rg_matrix(1,2)*2  Inductance=1e-3  SetiL0=off  InitialCurrent=0  Capacitance=Rg_matrix(1,2)*2  Setx0=off  InitialVoltage=0  Measurements=None
  Rcs*2 : powerlib/Elements/Series RLC Branch  LConnTagsString=__new0  RConnTagsString=__new0  BranchType=R  Resistance=-Rg_matrix(1,2)*2  Inductance=1e-3  SetiL0=off  InitialCurrent=0  Capacitance=Rg_matrix(1,2)*2  Setx0=off  InitialVoltage=0  Measurements=None
  Rgsg1/1 : powerlib/Elements/Series RLC Branch  LConnTagsString=__new0  RConnTagsString=__new0  BranchType=R  Resistance=(Rg_matrix(4,4)+Rg_matrix(3,4))*2  Inductance=1e-3  SetiL0=off  InitialCurrent=0  Capacitance=Rg_matrix(1,2)*2  Setx0=off  InitialVoltage=0  Measurements=None
  Rgsg1/2 : powerlib/Elements/Series RLC Branch  LConnTagsString=__new0  RConnTagsString=__new0  BranchType=R  Resistance=(Rg_matrix(2,2)+Rg_matrix(1,2))*2  Inductance=1e-3  SetiL0=off  InitialCurrent=0  Capacitance=Rg_matrix(1,2)*2  Setx0=off  InitialVoltage=0  Measurements=None
  Rgsg1/3 : powerlib/Elements/Series RLC Branch  LConnTagsString=__new0  RConnTagsString=__new0  BranchType=R  Resistance=(Rg_matrix(4,4)+Rg_matrix(3,4))*2  Inductance=1e-3  SetiL0=off  InitialCurrent=0  Capacitance=Rg_matrix(1,2)*2  Setx0=off  InitialVoltage=0  Measurements=None
  Rgsg1/4 : powerlib/Elements/Series RLC Branch  LConnTagsString=__new0  RConnTagsString=__new0  BranchType=R  Resistance=(Rg_matrix(2,2)+Rg_matrix(1,2))*2  Inductance=1e-3  SetiL0=off  InitialCurrent=0  Capacitance=Rg_matrix(1,2)*2  Setx0=off  InitialVoltage=0  Measurements=None
  Rsg*1 : powerlib/Elements/Series RLC Branch  LConnTagsString=__new0  RConnTagsString=__new0  BranchType=R  Resistance=(Rg_matrix(6,6)+Rg_matrix(5,6))*2  Inductance=1e-3  SetiL0=off  InitialCurrent=0  Capacitance=Rg_matrix(1,2)*2  Setx0=off  InitialVoltage=0  Measurements=None
  Rsg*2 : powerlib/Elements/Series RLC Branch  LConnTagsString=__new0  RConnTagsString=__new0  BranchType=R  Resistance=(Rg_matrix(6,6)+Rg_matrix(5,6))*2  Inductance=1e-3  SetiL0=off  InitialCurrent=0  Capacitance=Rg_matrix(1,2)*2  Setx0=off  InitialVoltage=0  Measurements=None
  A : PMIOPort  Side=Left
  B : PMIOPort  Port=2  Side=Left
  C : PMIOPort  Port=3  Side=Left
  a : PMIOPort  Port=4  Side=Right
  b : PMIOPort  Port=5  Side=Right
  c : PMIOPort  Port=6  Side=Right
  connections:
  A/RConn1 -- DPL/LConn1 -- Rcs*2/RConn1
  B/RConn1 -- DPL/LConn3 -- Ccs2/3/RConn1
  C/RConn1 -- DPL/LConn5 -- Ccs3/3/RConn1
  Rgsg1/2/RConn1 -- Rsg*2/RConn1 -- Rgsg1/1/RConn1 -- Ground2/LConn1
  DPL/LConn2 -- Rcs*2/LConn1 -- Rgsg1/2/LConn1 -- DPL/LConn4 -- Ccs2/3/LConn1 -- Rgsg1/1/LConn1 -- DPL/LConn6 -- Rsg*2/LConn1 -- Ccs3/3/LConn1 -- Ground3/LConn1
  Rgsg1/3/RConn1 -- Rsg*1/RConn1 -- Rgsg1/4/RConn1 -- Ground1/LConn1
  Rgsg1/3/LConn1 -- Ccs2/1/LConn1 -- DPL/RConn4 -- DPL/RConn2 -- Rgsg1/4/LConn1 -- Rcs*1/LConn1 -- Rsg*1/LConn1 -- Ccs3/1/LConn1 -- DPL/RConn6 -- Ground4/LConn1
  Rcs*1/RConn1 -- DPL/RConn1 -- a/RConn1
  DPL/RConn3 -- Ccs2/1/RConn1 -- b/RConn1
  DPL/RConn5 -- Ccs3/1/RConn1 -- c/RConn1
